simulink model "nl_offsets"  (Simulink 6.0)
settings: Solver=ode45  StartTime=0.0  StopTime=10.0  RelTol=1e-3
settings Model: LastModifiedBy=Alberto Bemporad  ExtModeTrigMode=oneshot  ExtModeArmWhenConnect=off
settings DataIOCC: LimitDataPoints=off  SignalLoggingName=logsOut
settings OptimizationCC: BooleanDataType=off
settings DebuggingCC: CheckExecutionContextPreStartOutputMsg=on  CheckExecutionContextRuntimeOutputMsg=on  SolverPrmCheckMsg=none
settings HardwareCC: TargetUnknown=on
settings SFSimCC: SFSimApplyToAllLibs=on  SFSimBuildMode=Incremental

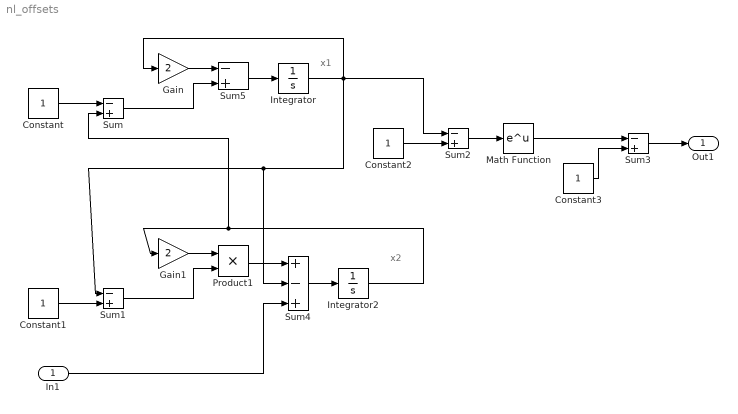
== system nl_offsets ==
  note: x1
  note: x2
  In1 : Inport  LatchInput=off
  Constant{,1..3} (4 alike) : Constant
  Gain : Gain  Gain=2  SaturateOnIntegerOverflow=on
  Gain1 : Gain  Gain=2  SaturateOnIntegerOverflow=on
  Integrator : Integrator  InitialCondition=0.7
  Integrator2 : Integrator  InitialCondition=1
  Math Function : Math  SaturateOnIntegerOverflow=on
  Product1 : Product  SaturateOnIntegerOverflow=on  RndMeth=Zero  InputSameDT=on
  Sum{,1..3,5} (5 alike) : Sum  Inputs=-+  SaturateOnIntegerOverflow=on  InputSameDT=on
  Sum4 : Sum  Inputs=+-+  SaturateOnIntegerOverflow=on  InputSameDT=on
  Out1 : Outport
  wires:
  Sum5/1 -> Integrator/1
  Gain/1 -> Sum5/1
  Integrator/1 -> Gain/1, Sum2/1, Sum1/1, Sum4/2
  Constant/1 -> Sum/1
  Sum/1 -> Sum5/2
  Gain1/1 -> Product1/1
  Sum1/1 -> Product1/2
  Constant1/1 -> Sum1/2
  Constant2/1 -> Sum2/2
  Sum2/1 -> Math Function/1
  Constant3/1 -> Sum3/2
  Math Function/1 -> Sum3/1
  Sum3/1 -> Out1/1
  Integrator2/1 -> Gain1/1, Sum/2
  Sum4/1 -> Integrator2/1
  Product1/1 -> Sum4/1
  In1/1 -> Sum4/3
